simulink model "Learning_project_3"  (R2021a)
settings: Solver=VariableStepAuto  StartTime=0.0  StopTime=100  MaxStep=0.01  RelTol=1e-3
settings Model: Creator=tanmoyera  LastModifiedBy=tanmoyera

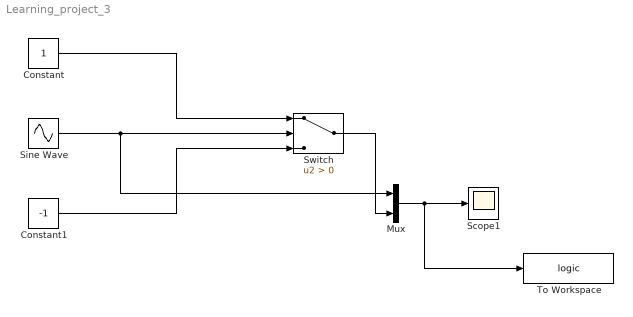
== system Learning_project_3 ==
  Constant : Constant
  Constant1 : Constant  Value=-1
  Mux : Mux  Inputs=2
  Scope1 : Scope
  Sine Wave : Sin  SampleTime=0
  Switch : Switch  Criteria=u2 > Threshold
  To Workspace : ToWorkspace  VariableName=logic  SaveFormat=Timeseries  SampleTime=-1
  wires:
  Sine Wave/1 -> Mux/1, Switch/2
  Constant/1 -> Switch/1
  Constant1/1 -> Switch/3
  Switch/1 -> Mux/2
  Mux/1 -> To Workspace/1, Scope1/1
